simulink model "Exp50x5B10x5D"  (R2024a)
settings: Solver=FixedStepAuto  StartTime=0.0  StopTime=10  FixedStep=0.01  RelTol=1e-3
libraries: spsDiodeLib x2, spsIGBTLib x2, spsDCVoltageSourceLib x1, spsCurrentMeasurementLib x1, spsDCMachineLib x1, spspowerguiLib x1, spsVoltageMeasurementLib x1, spsMultimeterLib x1
settings Model: Creator=srika  LastModifiedBy=kumar
settings DebuggingCC: UnconnectedInputMsg=warning  UnconnectedOutputMsg=warning  UnconnectedLineMsg=warning
settings ModelReferenceCC: EnableRefExpFcnMdlSchedulingChecks=on
settings RTWCC: GPUComputeCapability=3.5  DLArmComputeVersion=19.05

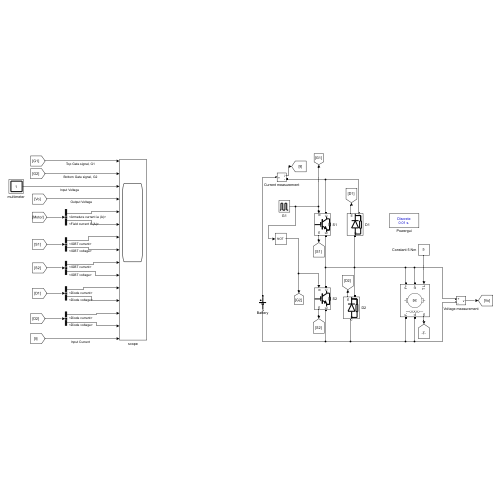
[thumbnail: Simulink's stored preview of the top-level diagram]
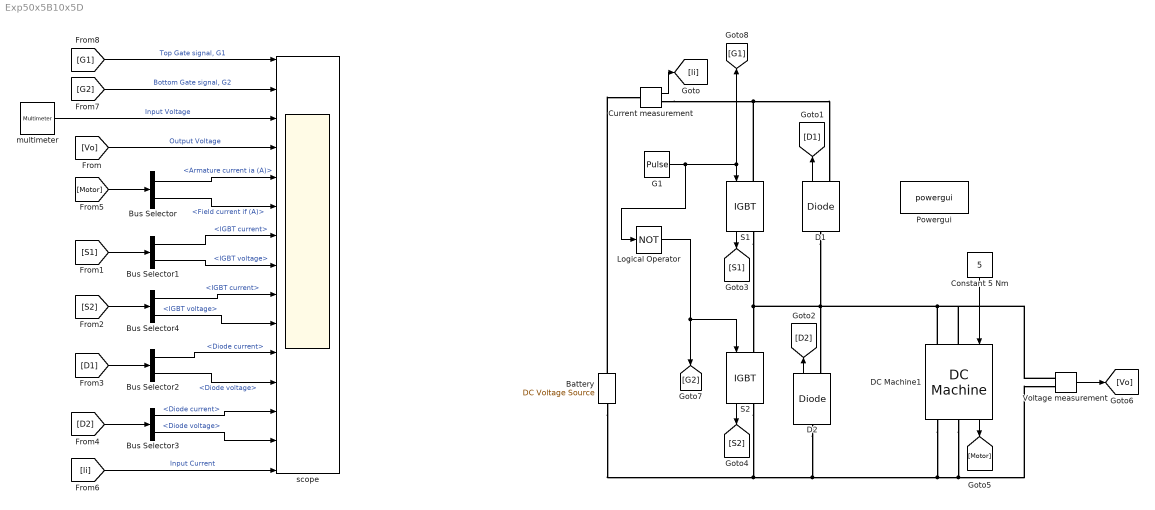
== system Exp50x5B10x5D ==
  Battery : spsDCVoltageSourceLib/DC Voltage Source  Amplitude=230  Measurements=Voltage
  Bus Selector : BusSelector  OutputSignals=Armature current ia (A),Field current if (A)
  Bus Selector1 : BusSelector  OutputSignals=IGBT current,IGBT voltage
  Bus Selector2 : BusSelector  OutputSignals=Diode current,Diode voltage
  Bus Selector3 : BusSelector  OutputSignals=Diode current,Diode voltage
  Bus Selector4 : BusSelector  OutputSignals=IGBT current,IGBT voltage
  Constant 5 Nm : Constant  Value=5
  Current measurement : spsCurrentMeasurementLib/Current Measurement  PhasorSimulation=off  OutputType=Complex  PSBequivalent=0
  D1 : spsDiodeLib/Diode  Ron=0.001  Lon=0  Vf=0.8  IC=0  UseSnubber=0  Rs=500  Cs=250e-9  Measurements=on
  D2 : spsDiodeLib/Diode  Ron=0.001  Lon=0  Vf=0.8  IC=0  UseSnubber=0  Rs=500  Cs=250e-9  Measurements=on
  DC Machine1 : spsDCMachineLib/DC Machine  PresetModel=No  MechanicalLoad=Torque TL  FieldType=Wound  ShowDetailedParameters=on  MeasurementBus=off  RLa="[ 0.6  0.012]"  RLf="[ 240  120]"  Laf=1.8  MachineConstant=Torque constant (N.m/A)  Ke=1.8  Kt=1.8  J=1  Bm=0  Tf=0  w0=1  Ifinit=5.73559215696593e-06  TsPowergui=0  TsBlock=-1
  G1 : DiscretePulseGenerator  PulseType=Time based  Period=4  PulseWidth=50
  Logical Operator : Logic  Operator=NOT  AllPortsSameDT=off  OutDataTypeStr=boolean
  Powergui : spspowerguiLib/powergui  Priority=1  SimulationMode=Discrete  SampleTime=1e-2  frequency=60  Iterations=50  frequencyindice=0  Pbase=100e6  ErrMax=1e-4  UnitsV=kV  UnitsW=MW  buscounter=0  FunctionMessages=off  echomessages=off  EnableUseOfTLC=off  CurrentSourceSwitches=off  DisableSnubberDevices=off  DisableRonSwitches=off  DisableVfSwitches=off  DisplayEquations=off  AutomaticDiscreteSolvers=off  SolverType=Tustin/Backward Euler (TBE)  Interpol=off  ExternalGateDelay=off  methode=off  Ts=100  x0status=blocks  SPID=on  SwTol=0  HookPort=off  NonlinearTolerance=1e-4  nMaxIteration=100  ContinueOnMaxIteration=off  RestoreLinks=warning  ResistiveCurrentMeasurement=off  Frange=[0:2:500]  Ylog=off  Xlog=on  ShowGrid=off  save=off  variable=ZData  structure=0  ZoomFFT=off  StartTime=0.0  cycles=1  DisplayStyle=1  fundamental=60  FreqAxis=off  MaxFrequency=1000  frequencyindicesteady=1  RmsSteady=1  display=off
  S1 : spsIGBTLib/IGBT  Ron=0.001  Lon=0  Vf=1  Tf=1e-6  Tt=2e-6  IC=0  Rs=1e5  Cs=inf  Measurements=on
  S2 : spsIGBTLib/IGBT  Ron=0.001  Lon=0  Vf=1  Tf=1e-6  Tt=2e-6  IC=0  Rs=1e5  Cs=inf  Measurements=on
  Voltage measurement : spsVoltageMeasurementLib/Voltage Measurement  PhasorSimulation=off  OutputType=Complex  PSBequivalent=0
  multimeter : spsMultimeterLib/Multimeter  L=1  sel=1  yselected={}  Gain=1  OutputType=Complex  PlotAtSimulationStop=off  PhasorSimulation=off
  scope : Scope  NumInputPorts=15
  wires:
  Constant 5 Nm/1 -> DC Machine1/1
  Voltage measurement/1 -> [Vo]
  DC Machine1/1 -> [Motor]
  Current measurement/1 -> [li]
  D2/1 -> [D2]
  S2/1 -> [S2]
  D1/1 -> [D1]
  S1/1 -> [S1]
  G1/1 -> Logical Operator/1, [G1], S1/1
  Logical Operator/1 -> [G2], S2/1
  [Motor] -> Bus Selector/1
  Bus Selector4/1 -> scope/9  "<IGBT current>"
  [G1] -> scope/1  "Top Gate signal, G1"
  [D1] -> Bus Selector2/1
  Bus Selector/2 -> scope/6  "<Field current if (A)>"
  [G2] -> scope/2  "Bottom Gate signal, G2"
  Bus Selector/1 -> scope/5  "<Armature current ia (A)>"
  [S2] -> Bus Selector4/1
  Bus Selector4/2 -> scope/10  "<IGBT voltage>"
  [D2] -> Bus Selector3/1
  multimeter/1 -> scope/3  "Input Voltage"
  Bus Selector3/1 -> scope/13  "<Diode current>"
  Bus Selector1/1 -> scope/7  "<IGBT current>"
  Bus Selector2/2 -> scope/12  "<Diode voltage>"
  [li] -> scope/15  "Input Current"
  [S1] -> Bus Selector1/1
  [Vo] -> scope/4  "Output Voltage"
  Bus Selector3/2 -> scope/14  "<Diode voltage>"
  Bus Selector2/1 -> scope/11  "<Diode current>"
  Bus Selector1/2 -> scope/8  "<IGBT voltage>"
  connections:
  Battery/RConn1 -- Current measurement/LConn1
  Battery/LConn1 -- S2/RConn1 -- DC Machine1/RConn2 -- DC Machine1/RConn1 -- Voltage measurement/LConn2 -- D2/LConn1
  Current measurement/RConn1 -- S1/LConn1 -- D1/RConn1
  D1/LConn1 -- DC Machine1/LConn2 -- DC Machine1/LConn1 -- Voltage measurement/LConn1 -- S2/LConn1 -- S1/RConn1 -- D2/RConn1
